simulink model "kavin"  (R2023b)
settings: Solver=VariableStepAuto  StartTime=0.0  StopTime=500  RelTol=1e-3
undefined symbols (not defined in the file or in its folder): alp_bet_v, omega_b, ptp, pulse, Vb
libraries: simulink x4, shared6dof x1, aerolibasang x1
settings Model: Creator=singh  LastModifiedBy=singh

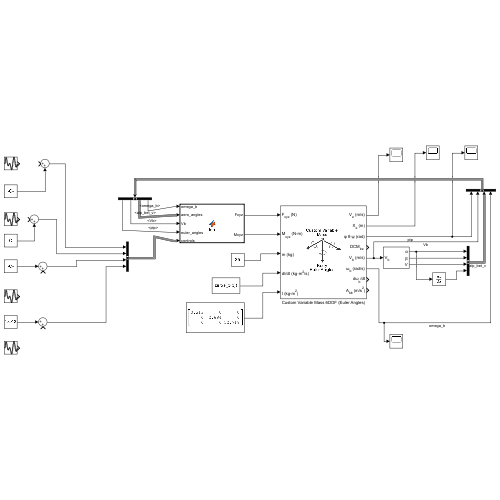
[thumbnail: Simulink's stored preview of the top-level diagram]
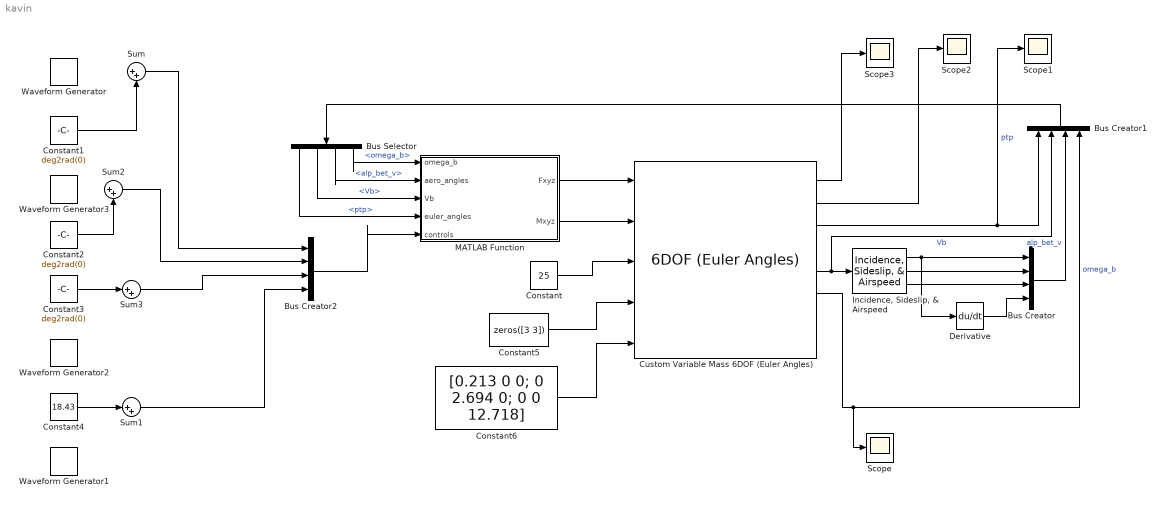
== system kavin ==
  Bus Creator : BusCreator  Inputs=4
  Bus Creator1 : BusCreator  Inputs=ptp,Vb,alp_bet_v,omega_b
  Bus Creator2 : BusCreator  Inputs=4
  Bus Selector : BusSelector  OutputSignals=ptp,Vb,alp_bet_v,omega_b
  Constant : Constant  Value=25
  Constant1 : Constant  Value=deg2rad(0)
  Constant2 : Constant  Value=deg2rad(0)
  Constant3 : Constant  Value=deg2rad(0)
  Constant4 : Constant  Value=18.43
  Constant5 : Constant  Value=zeros([3 3])
  Constant6 : Constant  Value=[0.213 0 0; 0 2.694 0; 0 0 12.718]
  Custom Variable Mass 6DOF (Euler Angles) : shared6dof/6DOF (Euler Angles)  units=Metric (MKS)  mtype=Custom Variable  rep=Euler Angles  xme_0=[0 0 0]  Vm_0=[43.25 0 0]  eul_0=[0 0 0]  pm_0=[0 0 0]  mass_0=1.0  mass_e=0.5  mass_f=2.0  inertia=eye(3)  inertia_e=eye(3)  inertia_f=2*eye(3)  k_quat=1.0  vre_flag=off  abi_flag=off  aMode=0  xme_statename=''  Vm_statename=''  eul_statename=''  quat_statename=''  pm_statename=''  mass_statename=''
      settings: LibrarySourceBlock=aerolib6dof2/Custom Variable Mass 6DOF (Euler Angles)
  Derivative : Derivative
  "Incidence, Sideslip, & Airspeed" : aerolibasang/Incidence, Sideslip, & Airspeed
  MATLAB Function : MATLAB Function  TreatAsAtomicUnit=on
  Scope{,1..3} (4 alike) : Scope
  Sum{,1..3} (4 alike) : Sum  Inputs=|++
  Waveform Generator : simulink/Sources/Waveform Generator  OutMin=[]  OutMax=[]  OutDataTypeStr=double  SelectedSignal=1  Signals=pulse('Amplitude',0.01,'TriggerTime',5,'Duration',1)  BlockNames=MultiportSwitch_bd3de8b3f62748b  SampleTime=0.1
  Waveform Generator1 : simulink/Sources/Waveform Generator  OutMin=[]  OutMax=[]  OutDataTypeStr=double  SelectedSignal=1  Signals=pulse('Amplitude',0.01,'TriggerTime',5,'Duration',1)  BlockNames=MultiportSwitch_16f4e64b5872446  SampleTime=0.1
  Waveform Generator2 : simulink/Sources/Waveform Generator  OutMin=[]  OutMax=[]  OutDataTypeStr=double  SelectedSignal=1  Signals=pulse('Amplitude',0.01,'TriggerTime',5,'Duration',1)  BlockNames=MultiportSwitch_bd3de8b3f62748b  SampleTime=0.1
  Waveform Generator3 : simulink/Sources/Waveform Generator  OutMin=[]  OutMax=[]  OutDataTypeStr=double  SelectedSignal=1  Signals=pulse('Amplitude',0.01,'TriggerTime',5,'Duration',1)  BlockNames=MultiportSwitch_bd3de8b3f62748b  SampleTime=0.1
  wires:
  MATLAB Function/1(Fxyz) -> Custom Variable Mass 6DOF (Euler Angles)/1
  MATLAB Function/2(Mxyz) -> Custom Variable Mass 6DOF (Euler Angles)/2
  Constant/1 -> Custom Variable Mass 6DOF (Euler Angles)/3
  Constant5/1 -> Custom Variable Mass 6DOF (Euler Angles)/4
  Constant6/1 -> Custom Variable Mass 6DOF (Euler Angles)/5
  Custom Variable Mass 6DOF (Euler Angles)/5 -> Bus Creator1/2, "Incidence, Sideslip, & Airspeed"/1  "Vb"
  "Incidence, Sideslip, & Airspeed"/1 -> Derivative/1, Bus Creator/1
  "Incidence, Sideslip, & Airspeed"/2 -> Bus Creator/2
  "Incidence, Sideslip, & Airspeed"/3 -> Bus Creator/3
  Derivative/1 -> Bus Creator/4
  Custom Variable Mass 6DOF (Euler Angles)/3 -> Scope1/1, Bus Creator1/1  "ptp"
  Bus Creator/1 -> Bus Creator1/3  "alp_bet_v"
  Custom Variable Mass 6DOF (Euler Angles)/6 -> Scope/1, Bus Creator1/4  "omega_b"
  Bus Creator1/1 -> Bus Selector/1
  Constant4/1 -> Sum1/1
  Sum1/1 -> Bus Creator2/4
  Constant1/1 -> Sum/2
  Sum/1 -> Bus Creator2/1
  Bus Creator2/1 -> MATLAB Function/5(controls)
  Custom Variable Mass 6DOF (Euler Angles)/1 -> Scope3/1
  Custom Variable Mass 6DOF (Euler Angles)/2 -> Scope2/1
  Bus Selector/1 -> MATLAB Function/4(euler_angles)  "<ptp>"
  Bus Selector/2 -> MATLAB Function/3(Vb)  "<Vb>"
  Bus Selector/3 -> MATLAB Function/2(aero_angles)  "<alp_bet_v>"
  Bus Selector/4 -> MATLAB Function/1(omega_b)  "<omega_b>"
  Sum2/1 -> Bus Creator2/2
  Constant3/1 -> Sum3/1
  Sum3/1 -> Bus Creator2/3
  Constant2/1 -> Sum2/2

== matlab function kavin/MATLAB Function ==
  data: omega_b input; Fxyz output; aero_angles input; Vb input; euler_angles input; controls input; Mxyz output
function [Fxyz,Mxyz] = fcn(omega_b, aero_angles, Vb, euler_angles, controls)
% Fxyz = [0 0 0];

g = 9.8; 
rho = 0.736; 
m = 25; 
C_bar = 0.431; 
b = 2.6; 
S_ref = 1.096;
C_L_0 = 0.14; 
C_L_alpha = 5.1; 
C_L_q = 3.825; 
C_L_delta_e = 0.65;
C_D_0 = 0.022; 
k = 0.06;
C_Y_beta = -0.223; 
C_Y_p = -0.104; 
C_Y_r = 0.151; 
C_Y_delta_a = 0;
C_l_beta = -0.0124;  
C_l_p = -0.3854; 
C_l_r = 0.16; 
C_l_delta_a = 0.24; 
C_l_delta_r = 0.0056;
C_M_0 = 0.03; 
C_M_alpha = -0.51; 
C_M_alpha_dot = -3.45; 
C_M_delta_e = -1.588;
C_N_beta = 0.055; 
C_N_p = -0.518; 
C_N_r = -0.067; 
C_N_delta_a = 0; 
C_N_delta_r = -0.031;

alpha = aero_angles(1);
beta = aero_angles(2);
V = aero_angles(3);
alpha_dot = aero_angles(4);

alpha_dot_hat = alpha_dot*C_bar/(2*V);

delta_e = controls(1);
delta_r = controls(2);
delta_a = controls(3);
delta_T = controls(4);

p = omega_b(1);
q = omega_b(2);
r = omega_b(3);

q_hat = q*C_bar/(2*V);

phi = euler_angles(1);
theta = euler_angles(2);
psi = euler_angles(3);

Q = 0.5*rho*V^2;

C_L = C_L_0 + C_L_alpha*alpha + C_L_delta_e*delta_e + C_L_q*q_hat;
C_D = C_D_0 + k*C_L^2;
C_Y = C_Y_beta*beta + C_Y_p*(p*b/(2*V)) + C_Y_r*(r*b/(2*V)) + C_Y_delta_a*delta_a;

C_l = C_l_beta*beta + C_l_p*(p*b/(2*V)) + C_l_r*(r*b/(2*V)) + C_l_delta_a*delta_a + C_l_delta_r*delta_r;
C_M = C_M_0 + C_M_alpha*alpha + C_M_delta_e*delta_e + C_M_alpha_dot*alpha_dot_hat;
C_N = C_N_beta*beta + C_N_p*(p*b/(2*V)) + C_N_r*(r*b/(2*V)) + C_N_delta_a*delta_a + C_N_delta_r*delta_r;

C_X = -C_D*cos(alpha) + C_L*sin(alpha);
C_Z = -C_D*sin(alpha) - C_L*cos(alpha);

Fx = delta_T + Q*C_X*S_ref - m*g*sin(theta);
Fy = Q*C_Y*S_ref;
Fz = Q*C_Z*S_ref + m*g*cos(theta);
Fxyz = [Fx; Fy; Fz];

Mx = Q*C_l*S_ref*b;
My = Q*C_M*S_ref*C_bar;
Mz = Q*C_N*S_ref*b;
Mxyz = [Mx; My; Mz];
